simulink model "RoverGPS"  (R2016b)
settings: Solver=ode3  StartTime=0.0  StopTime=30  RelTol=1e-3  EnableMultiTasking=on
undefined symbols (not defined in the file): Serial_Port, Standard_Devices
libraries: sldrtlib x2
settings Model: Creator=plopez  LastModifiedBy=Fakiko
settings DataIOCC: LimitDataPoints=on
settings OptimizationCC: LifeSpan=inf
settings DebuggingCC: SFUnexpectedBacktrackingDiag=warning  SFNoUnconditionalDefaultTransitionDiag=warning  SFExecutionAtInitializationDiag=none
settings HardwareCC: ProdBitPerSizeT=32  ProdBitPerPtrDiffT=32  ProdWordSize=32  ProdHWDeviceType=Specified
settings ModelReferenceCC: PropagateSignalLabelsOutOfModel=off
settings GRTTargetCC: TargetLangStandard=C89/C90 (ANSI)
settings ConfigComp: CovMetricSettings=dw  CovHtmlReporting=on  CovSaveCumulativeToWorkspaceVar=on  CovSaveSingleToWorkspaceVar=on  CovExternalEMLEnable=off

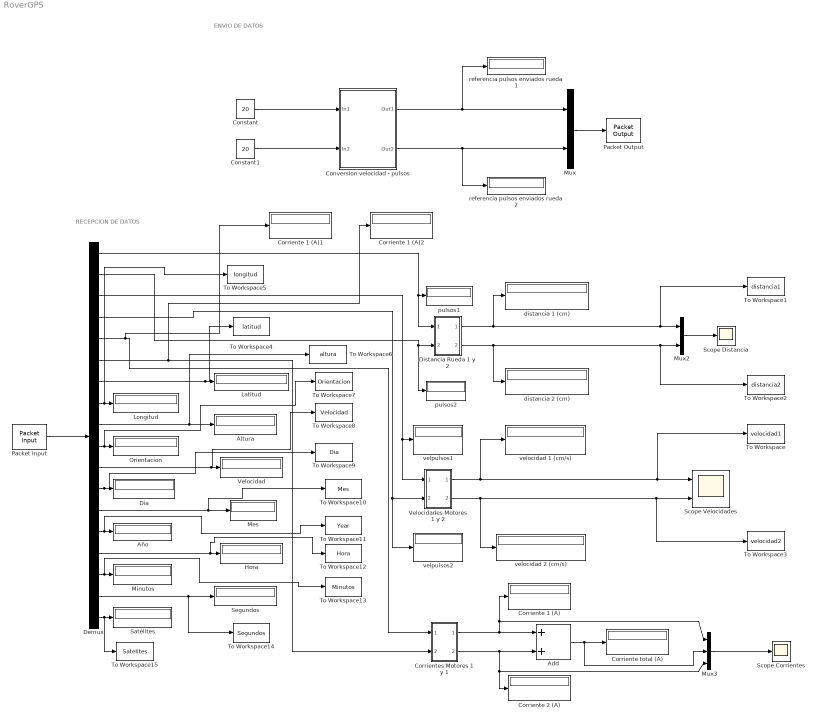
== system RoverGPS ==
  note: RECEPCION DE DATOS
  note: ENVIO DE DATOS
  Add : Sum
  Altura : Display
      settings: Format=decimal (Stored Integer)
  Año : Display
      settings: Format=decimal (Stored Integer)
  Constant : Constant  Value=20
  Constant1 : Constant  Value=20
  "Conversion velocidad - pulsos " : Subsystem
  Corriente 1 (A) : Display
      settings: Format=decimal (Stored Integer)
  Corriente 1 (A)1 : Display
      settings: Format=decimal (Stored Integer)
  Corriente 1 (A)2 : Display
      settings: Format=decimal (Stored Integer)
  Corriente 2 (A) : Display
      settings: Format=decimal (Stored Integer)
  Corriente total (A) : Display
      settings: Format=decimal (Stored Integer)
  Corrientes Motores 1 y 1 : Subsystem
  Demux : Demux  Outputs=18
  Dia : Display
      settings: Format=decimal (Stored Integer)
  "Distancia Rueda 1 y 2 " : Subsystem
  Hora : Display
      settings: Format=decimal (Stored Integer)
  Latitud : Display
      settings: Format=decimal (Stored Integer)
  Longitud : Display
      settings: Format=decimal (Stored Integer)
  Mes : Display
      settings: Format=decimal (Stored Integer)
  Minutos : Display
      settings: Format=decimal (Stored Integer)
  Mux : Mux  Inputs=2
  Mux2 : Mux  Inputs=2
  Mux3 : Mux  Inputs=3
  Orientacion : Display
      settings: Format=decimal (Stored Integer)
  Packet Input : sldrtlib/Packet Input  SampleTime=0.1  MaxMissedTicks=10  ShowMissedTicks=off  YieldWhenWaiting=off  DrvName=Standard_Devices/Serial_Port  DrvAddress=3  DrvOptions=[115200 8 0 0 0 0 0 0]  PacketSize=72  DataTypes='18*single'  ShowReady=off  ShowError=off  PacketID=1  ByteOrder=1  ShowTimestamp=off
      settings: AttributesFormatString=Serial Port [3]
  Packet Output : sldrtlib/Packet Output  SampleTime=0.1  MaxMissedTicks=10  ShowMissedTicks=off  YieldWhenWaiting=off  DrvName=Standard_Devices/Serial_Port  DrvAddress=3  DrvOptions=[115200 8 0 0 0 0 0 0]  PacketSize=4  DataTypes='2*int16'  ShowReady=off  ShowError=off  PacketID=1  ByteOrder=1  InitialValue=[]  FinalValue=[]
      settings: AttributesFormatString=Serial Port [3]
  Satélites : Display
      settings: Format=decimal (Stored Integer)
  Scope Corrientes : Scope
  Scope Distancia : Scope
  Scope Velocidades : Scope  NumInputPorts=2
  Segundos : Display
      settings: Format=decimal (Stored Integer)
  To Workspace : ToWorkspace  VariableName=velocidad1  SaveFormat=Structure With Time  SampleTime=-1
  To Workspace1 : ToWorkspace  VariableName=distancia1  SaveFormat=Structure With Time  SampleTime=-1
  To Workspace10 : ToWorkspace  VariableName=Mes  SaveFormat=Structure With Time  SampleTime=-1
  To Workspace11 : ToWorkspace  VariableName=Year  SaveFormat=Structure With Time  SampleTime=-1
  To Workspace12 : ToWorkspace  VariableName=Hora  SaveFormat=Structure With Time  SampleTime=-1
  To Workspace13 : ToWorkspace  VariableName=Minutos  SaveFormat=Structure With Time  SampleTime=-1
  To Workspace14 : ToWorkspace  VariableName=Segundos  SaveFormat=Structure With Time  SampleTime=-1
  To Workspace15 : ToWorkspace  VariableName=Satelites  SaveFormat=Structure With Time  SampleTime=-1
  To Workspace2 : ToWorkspace  VariableName=distancia2  SaveFormat=Structure With Time  SampleTime=-1
  To Workspace3 : ToWorkspace  VariableName=velocidad2  SaveFormat=Structure With Time  SampleTime=-1
  To Workspace4 : ToWorkspace  VariableName=latitud  SaveFormat=Structure With Time  SampleTime=-1
  To Workspace5 : ToWorkspace  VariableName=longitud  SaveFormat=Structure With Time  SampleTime=-1
  To Workspace6 : ToWorkspace  VariableName=altura  SaveFormat=Structure With Time  SampleTime=-1
  To Workspace7 : ToWorkspace  VariableName=Orientacion  SaveFormat=Structure With Time  SampleTime=-1
  To Workspace8 : ToWorkspace  VariableName=Velocidad  SaveFormat=Structure With Time  SampleTime=-1
  To Workspace9 : ToWorkspace  VariableName=Dia  SaveFormat=Structure With Time  SampleTime=-1
  Velocidad : Display
      settings: Format=decimal (Stored Integer)
  "Velocidades Motores 1 y 2 " : Subsystem
  distancia 1 (cm) : Display
      settings: Format=decimal (Stored Integer)
  distancia 2 (cm) : Display
      settings: Format=decimal (Stored Integer)
  pulsos1 : Display
      settings: Format=decimal (Stored Integer)
  pulsos2 : Display
      settings: Format=decimal (Stored Integer)
  "referencia pulsos enviados rueda 1 " : Display
      settings: Format=decimal (Stored Integer)  Decimation=2
  "referencia pulsos enviados rueda 2 " : Display
      settings: Format=decimal (Stored Integer)  Decimation=2
  velocidad 1 (cm/s) : Display
      settings: Format=decimal (Stored Integer)
  velocidad 2 (cm/s) : Display
      settings: Format=decimal (Stored Integer)
  velpulsos1 : Display
      settings: Format=decimal (Stored Integer)
  velpulsos2 : Display
      settings: Format=decimal (Stored Integer)
  wires:
  Demux/1 -> "Distancia Rueda 1 y 2 "/1(In1), pulsos1/1
  Demux/2 -> pulsos2/1, "Distancia Rueda 1 y 2 "/2(In2)
  Packet Input/1 -> Demux/1
  Demux/3 -> "Velocidades Motores 1 y 2 "/1(In1), velpulsos1/1
  Demux/4 -> velpulsos2/1, "Velocidades Motores 1 y 2 "/2(In2)
  Mux/1 -> Packet Output/1
  Corrientes Motores 1 y 1/2(Out2) -> Add/2, Mux3/3, Corriente 2 (A)/1
  Demux/5 -> Corrientes Motores 1 y 1/1(In1), Corriente 1 (A)1/1
  Demux/6 -> Corrientes Motores 1 y 1/2(In2), Corriente 1 (A)2/1
  "Distancia Rueda 1 y 2 "/1(Out1) -> Mux2/1, To Workspace1/1, distancia 1 (cm)/1
  "Distancia Rueda 1 y 2 "/2(Out2) -> To Workspace2/1, Mux2/2, distancia 2 (cm)/1
  "Conversion velocidad - pulsos "/1(Out1) -> "referencia pulsos enviados rueda 1 "/1, Mux/1
  "Conversion velocidad - pulsos "/2(Out2) -> Mux/2, "referencia pulsos enviados rueda 2 "/1
  "Velocidades Motores 1 y 2 "/1(Out1) -> velocidad 1 (cm/s)/1, To Workspace/1, Scope Velocidades/1
  "Velocidades Motores 1 y 2 "/2(Out2) -> velocidad 2 (cm/s)/1, To Workspace3/1, Scope Velocidades/2
  Mux2/1 -> Scope Distancia/1
  Mux3/1 -> Scope Corrientes/1
  Corrientes Motores 1 y 1/1(Out1) -> Add/1, Corriente 1 (A)/1, Mux3/1
  Add/1 -> Mux3/2, Corriente total (A)/1
  Demux/8 -> To Workspace5/1, Longitud/1
  Demux/7 -> To Workspace4/1, Latitud/1
  Demux/9 -> To Workspace6/1, Altura/1
  Demux/12 -> To Workspace9/1, Dia/1
  Demux/13 -> Mes/1, To Workspace10/1
  Demux/14 -> To Workspace11/1, Año/1
  Demux/15 -> Hora/1, To Workspace12/1
  Demux/16 -> To Workspace13/1, Minutos/1
  Demux/17 -> Segundos/1, To Workspace14/1
  Demux/18 -> To Workspace15/1, Satélites/1
  Demux/10 -> To Workspace7/1, Orientacion/1
  Demux/11 -> To Workspace8/1, Velocidad/1
  Constant/1 -> "Conversion velocidad - pulsos "/1(In1)
  Constant1/1 -> "Conversion velocidad - pulsos "/2(In2)

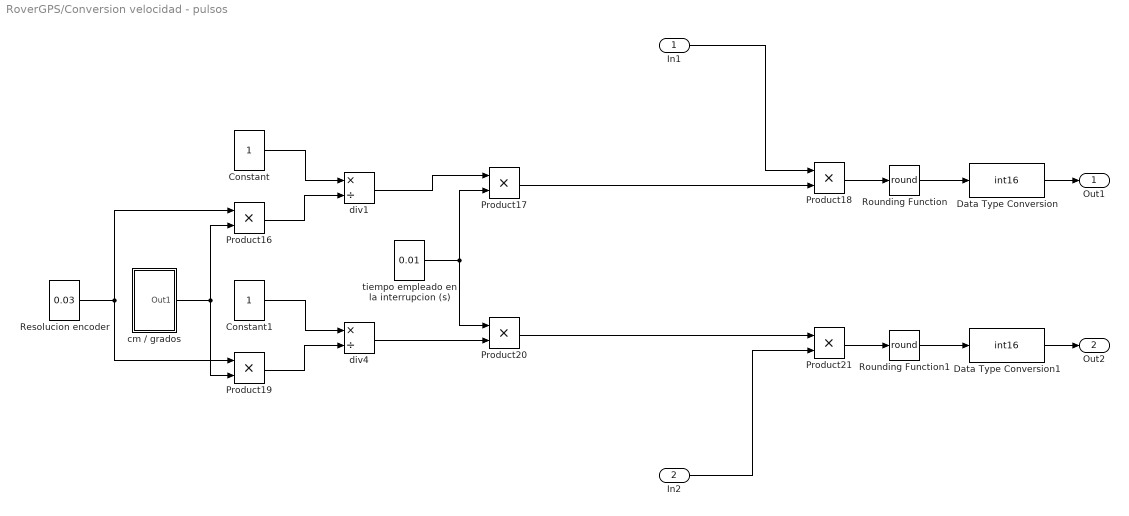
== system RoverGPS/Conversion velocidad - pulsos  ==
  In1 : Inport
  In2 : Inport  Port=2
  Constant : Constant
  Constant1 : Constant
  Data Type Conversion : DataTypeConversion  OutDataTypeStr=int16
  Data Type Conversion1 : DataTypeConversion  OutDataTypeStr=int16
  Product{16..21} (6 alike) : Product
  Resolucion encoder : Constant  Value=0.03
  Rounding Function : Rounding  Operator=round
  Rounding Function1 : Rounding  Operator=round
  cm / grados : Subsystem
  div1 : Product  Inputs=*/
  div4 : Product  Inputs=*/
  tiempo empleado en la interrupcion (s) : Constant  Value=0.01
  Out1 : Outport
  Out2 : Outport  Port=2
  wires:
  cm / grados/1(Out1) -> Product19/2, Product16/2
  div1/1 -> Product17/1
  In2/1 -> Product21/2
  Resolucion encoder/1 -> Product16/1, Product19/1
  Product16/1 -> div1/2
  Constant/1 -> div1/1
  tiempo empleado en la interrupcion (s)/1 -> Product17/2, Product20/1
  Product17/1 -> Product18/2
  In1/1 -> Product18/1
  Product19/1 -> div4/2
  Constant1/1 -> div4/1
  div4/1 -> Product20/2
  Product21/1 -> Rounding Function1/1
  Data Type Conversion/1 -> Out1/1
  Data Type Conversion1/1 -> Out2/1
  Product18/1 -> Rounding Function/1
  Rounding Function/1 -> Data Type Conversion/1
  Rounding Function1/1 -> Data Type Conversion1/1
  Product20/1 -> Product21/1

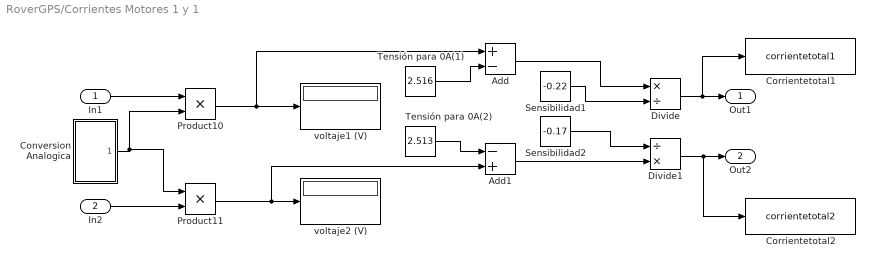
== system RoverGPS/Corrientes Motores 1 y 1 ==
  In1 : Inport
  In2 : Inport  Port=2
  Add : Sum  Inputs=+-
  Add1 : Sum  Inputs=-+
  Conversion Analogica : Subsystem
  Corrientetotal1 : ToWorkspace  VariableName=corrientetotal1  SaveFormat=Timeseries  SampleTime=-1
  Corrientetotal2 : ToWorkspace  VariableName=corrientetotal2  SaveFormat=Timeseries  SampleTime=-1
  Divide : Product  Inputs=*/
  Divide1 : Product  Inputs=/*
  Product10 : Product
  Product11 : Product
  Sensibilidad1 : Constant  Value=-0.22
  Sensibilidad2 : Constant  Value=-0.17
  "Tensión para 0A(1) " : Constant  Value=2.516
  Tensión para 0A(2) : Constant  Value=2.513
  voltaje1 (V) : Display
      settings: Format=decimal (Stored Integer)
  voltaje2 (V) : Display
      settings: Format=decimal (Stored Integer)
  Out1 : Outport
  Out2 : Outport  Port=2
  wires:
  In1/1 -> Product10/1
  Conversion Analogica/1(Tensión) -> Product11/1, Product10/2
  Product10/1 -> Add/1, voltaje1 (V)/1
  Product11/1 -> Add1/2, voltaje2 (V)/1
  "Tensión para 0A(1) "/1 -> Add/2
  Add/1 -> Divide/1
  Sensibilidad1/1 -> Divide/2
  Add1/1 -> Divide1/2
  Divide/1 -> Corrientetotal1/1, Out1/1
  Divide1/1 -> Corrientetotal2/1, Out2/1
  In2/1 -> Product11/2
  Tensión para 0A(2)/1 -> Add1/1
  Sensibilidad2/1 -> Divide1/1

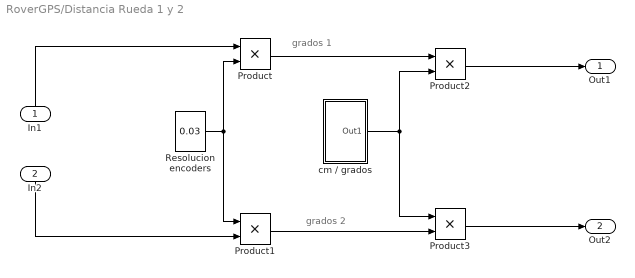
== system RoverGPS/Distancia Rueda 1 y 2  ==
  note: grados 2
  note: grados 1
  In1 : Inport
  In2 : Inport  Port=2
  Product{,1..3} (4 alike) : Product
  Resolucion encoders : Constant  Value=0.03
  "cm / grados " : Subsystem
  Out1 : Outport
  Out2 : Outport  Port=2
  wires:
  "cm / grados "/1(Out1) -> Product2/2, Product3/1
  Resolucion encoders/1 -> Product/2, Product1/1
  In1/1 -> Product/1
  In2/1 -> Product1/2
  Product/1 -> Product2/1
  Product1/1 -> Product3/2
  Product2/1 -> Out1/1
  Product3/1 -> Out2/1

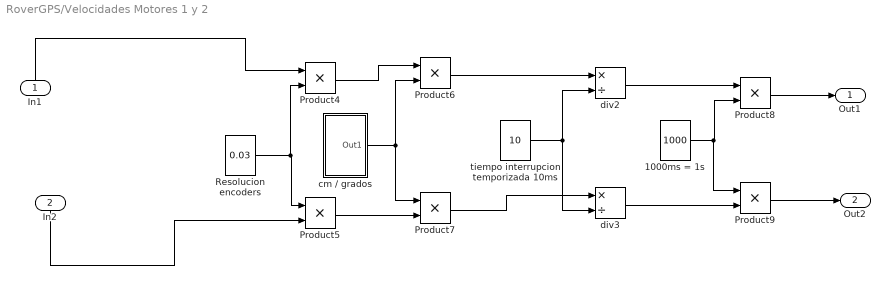
== system RoverGPS/Velocidades Motores 1 y 2  ==
  In1 : Inport
  In2 : Inport  Port=2
  1000ms = 1s : Constant  Value=1000
  Product{4..9} (6 alike) : Product
  Resolucion encoders : Constant  Value=0.03
  cm / grados : Subsystem
  div2 : Product  Inputs=*/
  div3 : Product  Inputs=*/
  tiempo interrupcion temporizada 10ms : Constant  Value=10
  Out1 : Outport
  Out2 : Outport  Port=2
  wires:
  cm / grados/1(Out1) -> Product7/1, Product6/2
  Product4/1 -> Product6/1
  In1/1 -> Product4/1
  Resolucion encoders/1 -> Product4/2, Product5/1
  In2/1 -> Product5/2
  Product5/1 -> Product7/2
  Product6/1 -> div2/1
  tiempo interrupcion temporizada 10ms/1 -> div3/2, div2/2
  div2/1 -> Product8/1
  div3/1 -> Product9/2
  1000ms = 1s/1 -> Product9/1, Product8/2
  Product8/1 -> Out1/1
  Product9/1 -> Out2/1
  Product7/1 -> div3/1

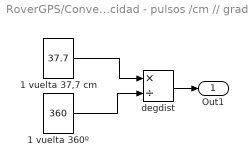
== system RoverGPS/Conversion velocidad - pulsos /cm // grados ==
  1 vuelta 360º : Constant  Value=360
  1 vuelta 37,7 cm : Constant  Value=37.7
  degdist : Product  Inputs=*/
  Out1 : Outport
  wires:
  1 vuelta 37,7 cm/1 -> degdist/1
  1 vuelta 360º/1 -> degdist/2
  degdist/1 -> Out1/1

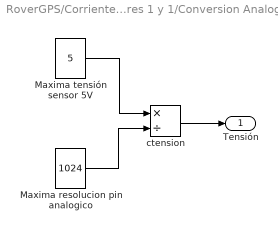
== system RoverGPS/Corrientes Motores 1 y 1/Conversion Analogica ==
  "Maxima resolucion pin analogico " : Constant  Value=1024
  Maxima tensión sensor 5V : Constant  Value=5
  ctension : Product  Inputs=*/
  Tensión : Outport
  wires:
  Maxima tensión sensor 5V/1 -> ctension/1
  "Maxima resolucion pin analogico "/1 -> ctension/2
  ctension/1 -> Tensión/1

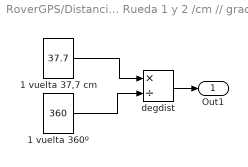
== system RoverGPS/Distancia Rueda 1 y 2 /cm // grados  ==
  1 vuelta 360º : Constant  Value=360
  1 vuelta 37,7 cm : Constant  Value=37.7
  degdist : Product  Inputs=*/
  Out1 : Outport
  wires:
  1 vuelta 37,7 cm/1 -> degdist/1
  1 vuelta 360º/1 -> degdist/2
  degdist/1 -> Out1/1

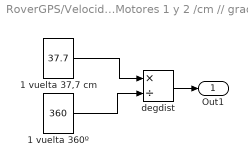
== system RoverGPS/Velocidades Motores 1 y 2 /cm // grados ==
  1 vuelta 360º : Constant  Value=360
  1 vuelta 37,7 cm : Constant  Value=37.7
  degdist : Product  Inputs=*/
  Out1 : Outport
  wires:
  1 vuelta 37,7 cm/1 -> degdist/1
  1 vuelta 360º/1 -> degdist/2
  degdist/1 -> Out1/1
